simulink model "controlador_malha_fechada_integral_21_a"  (R2021a)
settings: Solver=ode4  StartTime=0.0  StopTime=2  RelTol=1e-3
values from neighbouring files (symbols this model uses):
  K_barra = 1    [closed_loop_integral_parameters.m]
  Ki = zeros(4,1)    [closed_loop_integral_parameters.m]
undefined symbols (not defined in the file or in its folder): Ka, Kt, tau
settings Model: Creator=Guilherme  LastModifiedBy=Guilherme
settings DebuggingCC: UnconnectedInputMsg=none  UnconnectedOutputMsg=none  UnconnectedLineMsg=none
settings ModelReferenceCC: EnableRefExpFcnMdlSchedulingChecks=off
settings RTWCC: Description=Generic Real-Time Target  GPUComputeCapability=5.0  DLArmComputeVersion=20.02.1

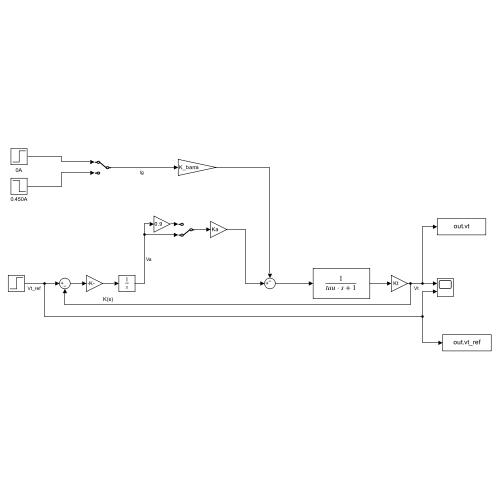
[thumbnail: Simulink's stored preview of the top-level diagram]
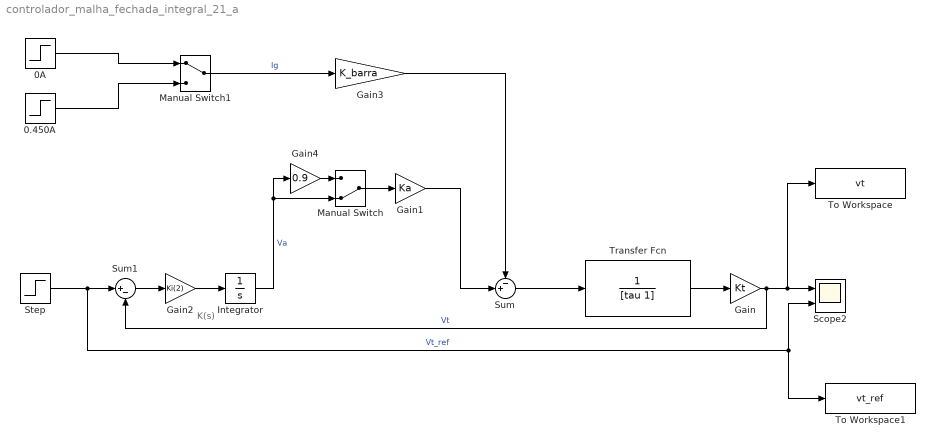
== system controlador_malha_fechada_integral_21_a ==
  note: K(s)
  0.450A : Step  Time=0  Before=0.450  After=0  SampleTime=0
  0A : Step  Time=0  After=0  SampleTime=0
  Gain : Gain  Gain=Kt
  Gain1 : Gain  Gain=Ka
  Gain2 : Gain  Gain=Ki(2)
  Gain3 : Gain  Gain=K_barra
  Gain4 : Gain  Gain=0.9
  Integrator : Integrator
  Manual Switch : ManualSwitch  CurrentSetting=0
  Manual Switch1 : ManualSwitch
  Scope2 : Scope  NumInputPorts=2
  Step : Step  Time=0  After=10  SampleTime=0
  Sum : Sum  Inputs=-+|
  Sum1 : Sum  Inputs=|+-
  To Workspace : ToWorkspace  VariableName=vt  SaveFormat=Timeseries  SampleTime=-1
  To Workspace1 : ToWorkspace  VariableName=vt_ref  SaveFormat=Timeseries  SampleTime=-1
  Transfer Fcn : TransferFcn  Denominator=[tau 1]
  wires:
  Gain3/1 -> Sum/1
  Sum/1 -> Transfer Fcn/1
  Manual Switch/1 -> Gain1/1
  Gain4/1 -> Manual Switch/1
  Gain1/1 -> Sum/2
  Gain/1 -> Sum1/2, To Workspace/1, Scope2/1  "Vt"
  Transfer Fcn/1 -> Gain/1
  Step/1 -> Scope2/2, To Workspace1/1, Sum1/1  "Vt_ref"
  Sum1/1 -> Gain2/1
  Gain2/1 -> Integrator/1
  Integrator/1 -> Manual Switch/2, Gain4/1  "Va"
  Manual Switch1/1 -> Gain3/1  "Ig"
  0A/1 -> Manual Switch1/1
  0.450A/1 -> Manual Switch1/2
